simulink model "Teorico_Real"  (R2023b)
settings: Solver=VariableStepAuto  StartTime=0.0  StopTime=10.0  RelTol=1e-3
InitFcn:
  | R=5.2;
  | L=9.38e-4;
  | J=0.0072;
  | B=3.89e-4;
  | Ra=0.05;
  | km=0.5931;
settings Model: Creator=marqu  LastModifiedBy=marqu

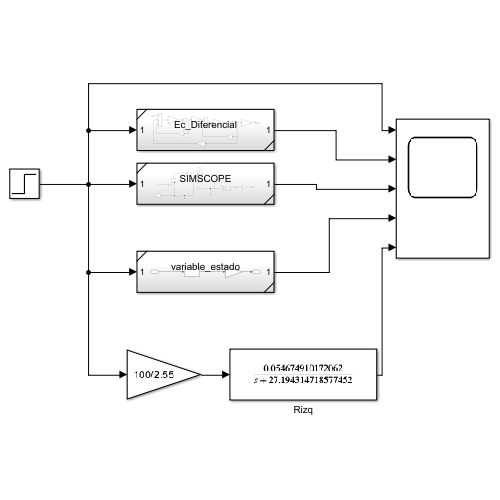
[thumbnail: Simulink's stored preview of the top-level diagram]
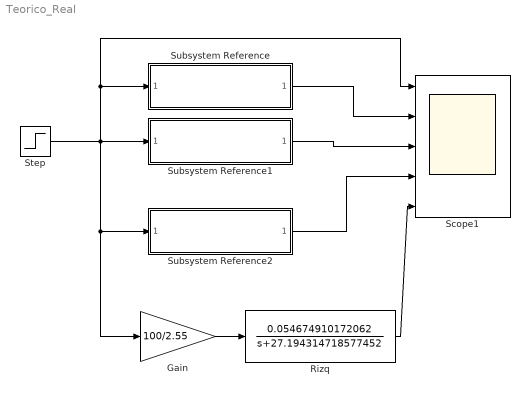
== system Teorico_Real ==
  Gain : Gain  Gain=100/2.55
  Rizq : TransferFcn  Numerator=[0.054674910172062]  Denominator=[1,27.194314718577452]
  Scope1 : Scope  NumInputPorts=5
  Step : Step  After=0.5  SampleTime=0
  Subsystem Reference : Subsystem  ReferencedSubsystem=Ec_Diferencial
  Subsystem Reference1 : Subsystem  ReferencedSubsystem=SIMSCOPE
  Subsystem Reference2 : Subsystem  ReferencedSubsystem=variable_estado
  wires:
  Subsystem Reference2/1 -> Scope1/4
  Subsystem Reference1/1 -> Scope1/3
  Subsystem Reference/1 -> Scope1/2
  Step/1 -> Subsystem Reference/1, Scope1/1, Subsystem Reference1/1, Gain/1, Subsystem Reference2/1
  Rizq/1 -> Scope1/5
  Gain/1 -> Rizq/1
